simulink model "ModeInt"  (R2018b)
settings: Solver=FixedStepDiscrete  StartTime=0.0  StopTime=10.0  FixedStep=0.01  RelTol=1e-3
undefined symbols (not defined in the file or in its folder): c, CmprtMdHMIReqTp1, e, IfVeSMSeStNumConfig, MdReqTp1
(part 3 of 4)

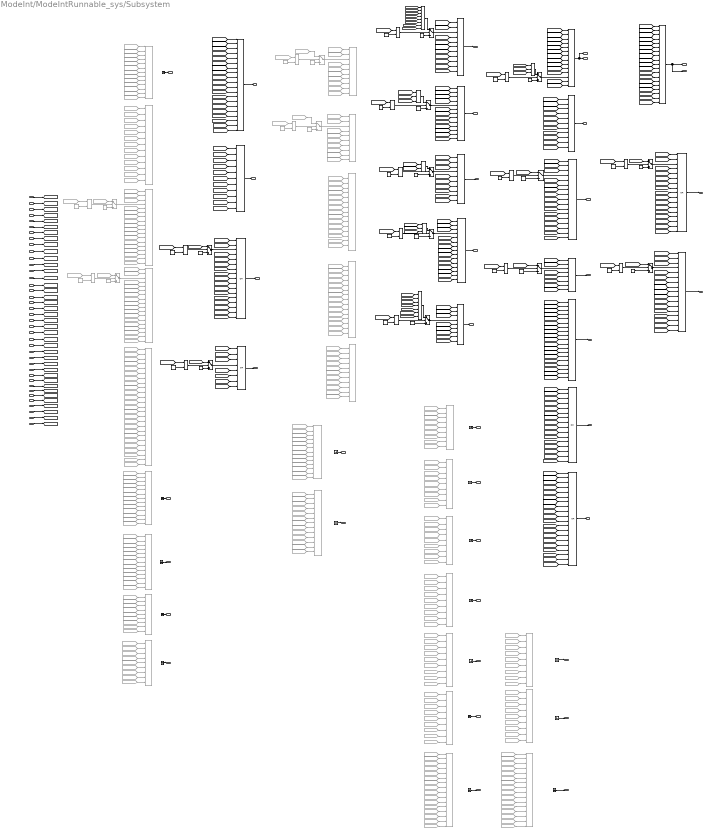
== system ModeInt/ModeIntRunnable_sys/Subsystem ==
  note: 2022-02-17:CR202175：修改需求506/548/551/552，新增需求712，完善座椅模式的打断策略。
  acsExtSoftInt : Inport
  acsEntySoftInt : Inport  Port=2
  LtVipSoftInt : Inport  Port=3
  RtVipSoftInt : Inport  Port=4
  LtLugSoftInt : Inport  Port=5
  RtLugSoftInt : Inport  Port=6
  AllLugSoftInt : Inport  Port=7
  LtRcvySoftInt : Inport  Port=8
  RtRcvySoftInt : Inport  Port=9
  SeStNumConfig : Inport  Port=10
  AllVipSoftInt : Inport  Port=11
  LtFamilySoftInt : Inport  Port=12
  RtFamilySoftInt : Inport  Port=13
  IntimacyLtSoftInt : Inport  Port=14
  IntimacyRtSoftInt : Inport  Port=15
  LtLyingSoftInt : Inport  Port=16
  RtLyingSoftInt : Inport  Port=17
  LgrstOpenLtSoftInt : Inport  Port=18
  LgrstCloseLtSoftInt : Inport  Port=19
  LgrstOpenRtSoftInt : Inport  Port=20
  LgrstCloseRtSoftInt : Inport  Port=21
  acsEntry4s2LSoftInt : Inport  Port=22
  " acsEntry4s2RSoftInt" : Inport  Port=23
  acsExit4s2LSoftInt : Inport  Port=24
  acsExit4s2RSoftInt : Inport  Port=25
  acsEntryAll4sBwdSoftInt : Inport  Port=26
  acsEntryAll4sFwdSoftInt : Inport  Port=27
  PasReclinerEntrySoftInt : Inport  Port=28
  PasReclinerExitSoftInt : Inport  Port=29
  VIPLtOutSoftInt : Inport  Port=30
  VIPRtOutSoftInt : Inport  Port=31
  VIPAllOutSoftInt : Inport  Port=32
  Big4SeatSoftInt : Inport  Port=33
  Unfold3LSoftInt : Inport  Port=34
  Unfold3RSoftInt : Inport  Port=35
  ExVIPRSoftInt : Inport  Port=36
  ExVIPROutSoftInt : Inport  Port=37
  WholeVehMem1SoftInt : Inport  Port=38
  WholeVehMem2SoftInt : Inport  Port=39
  Constant{1,3,5,7} (4 alike) : Constant  Commented=on  Value=IfVeSMSeStNumConfig.SeatNum7Config  OutDataTypeStr=Enum: IfVeSMSeStNumConfig
  Constant{10,12,14,16,18,20,22,24,26,28,30,32} (12 alike) : Constant  Value=0  OutDataTypeStr=uint8
  Constant{9,11,13,15,17,19,21,23,25,27,29,31} (12 alike) : Constant  Value=IfVeSMSeStNumConfig.SeatNum7Config  OutDataTypeStr=Enum: IfVeSMSeStNumConfig
  Constant{2,4,6,8} (4 alike) : Constant  Commented=on  Value=0  OutDataTypeStr=uint8
  Equal{1..4} (4 alike) : RelationalOperator  Commented=on  Operator===  OutDataTypeStr=boolean  RndMeth=Simplest
  Equal{5..16} (12 alike) : RelationalOperator  Operator===  OutDataTypeStr=boolean  RndMeth=Simplest
  From{,164,200,204,236,297,306,320,336} (9 alike) : From  Commented=on  GotoTag=LgrstOpenRtSoftInt
  From{1,6,16,22,27,31,34,37,87,99,119,131,170} (13 alike) : From  Commented=on  GotoTag=acsEntySoftInt
  From{10,17,23,43,138,155,181,185,194,197} (10 alike) : From  Commented=on  GotoTag=LtLugSoftInt
  From{2,8,28,32,38,88,97,100,109,120,122,146,206,228,275,284,311,327} (18 alike) : From  Commented=on  GotoTag=LtVipSoftInt
  From{3,9,29,35,39,42,101,110,136,147,171,180,216,240,293,302,313,328} (18 alike) : From  Commented=on  GotoTag=RtVipSoftInt
  From{4,13,20,91,102,111,123,150,172,177,235,277,286,314,330} (15 alike) : From  Commented=on  GotoTag=LtRcvySoftInt
  From{5,14,26,90,103,112,137,151,173,223,247,295,304,315,331} (15 alike) : From  Commented=on  GotoTag=RtRcvySoftInt
  From{47,53,67..70,73,76,81,93,104,113,174,205,207..208,210..212,276,285,294,303,312,329} (25 alike) : From  Commented=on  GotoTag=AllVipSoftInt
  From{55,75,79,84,105,114,145,148,154,156,158,162,188} (13 alike) : From  Commented=on  GotoTag=IntimacyLtSoftInt
  From{49,54,58,62,66,72,78,83,95,106,128,144,176} (13 alike) : From  Commented=on  GotoTag=RtFamilySoftInt
  From{50,59,96,107,125,149,157,159,163,167,179,184,189} (13 alike) : From  Commented=on  GotoTag=IntimacyRtSoftInt
  From{48,57,61,65,71,77,82,94,108,115,127,143,175} (13 alike) : From  Commented=on  GotoTag=LtFamilySoftInt
  From{11,18,24,45,139,153,182,186,195,198} (10 alike) : From  Commented=on  GotoTag=RtLugSoftInt
  From{36,40,44,117} (4 alike) : From  Commented=on  GotoTag=SeStNumConfig
  From{7,15,21,30,33,41,52,86,92,98,118,130,152} (13 alike) : From  Commented=on  GotoTag=acsExtSoftInt
  From{12,19,25,46,74,124,140,183,187,196,199} (11 alike) : From  Commented=on  GotoTag=AllLugSoftInt
  From{126,134,168,218,226,232,239,246,250,254,258,282,291,300,309,342} (16 alike) : From  Commented=on  GotoTag=acsEntryAll4sBwdSoftInt
  From{129,135,169,220,227,233,241,245,251,255,259,283,292,301,310,325} (16 alike) : From  Commented=on  GotoTag=acsEntryAll4sFwdSoftInt
  From{132,213,221,234,248,252,290,322,338} (9 alike) : From  Commented=on  GotoTag=acsEntry4s2LSoftInt
  From{133,214,222,238,249,253,281,324,340} (9 alike) : From  Commented=on  GotoTag=acsExit4s2LSoftInt
  From{141,215,229,242,256,260,308,323,339} (9 alike) : From  Commented=on  GotoTag=acsEntry4s2RSoftInt
  From{142,217,230,244,257,261,299,326,341} (9 alike) : From  Commented=on  GotoTag=acsExit4s2RSoftInt
  From{63,160,192,202,225,279,288,318,334} (9 alike) : From  Commented=on  GotoTag=LgrstOpenLtSoftInt
  From{161,166,193,203,224,280,289,319,335} (9 alike) : From  Commented=on  GotoTag=LgrstCloseLtSoftInt
  From{89,165,191,201,237,298,307,321,337} (9 alike) : From  Commented=on  GotoTag=LgrstCloseRtSoftInt
  From{60,80,178,209,231,278,287,316,332} (9 alike) : From  Commented=on  GotoTag=LtLyingSoftInt
  From{64,85,190,219,243,296,305,317,333} (9 alike) : From  Commented=on  GotoTag=RtLyingSoftInt
  Ground{,1..16} (17 alike) : Ground
  OR{,1,9..11,15} (6 alike) : Logic  Commented=on  Operator=OR  Inputs=13  AllPortsSameDT=off  OutDataTypeStr=boolean
  OR{12..13,16..23} (10 alike) : Logic  Commented=on  Operator=OR  Inputs=9  AllPortsSameDT=off  OutDataTypeStr=boolean
  OR14 : Logic  Commented=on  Operator=OR  Inputs=25  AllPortsSameDT=off  OutDataTypeStr=boolean
  OR2 : Logic  Commented=on  Operator=OR  Inputs=18  AllPortsSameDT=off  OutDataTypeStr=boolean
  OR24 : Logic  Commented=on  Operator=OR  Inputs=16  AllPortsSameDT=off  OutDataTypeStr=boolean
  OR25 : Logic  Commented=on  Operator=OR  Inputs=16  AllPortsSameDT=off  OutDataTypeStr=boolean
  OR26 : Logic  Operator=OR  Inputs=20  AllPortsSameDT=off  OutDataTypeStr=boolean
  OR27 : Logic  Operator=OR  Inputs=11  AllPortsSameDT=off  OutDataTypeStr=boolean
  OR28 : Logic  Operator=OR  Inputs=19  AllPortsSameDT=off  OutDataTypeStr=boolean
  OR{29,43,46..47} (4 alike) : Logic  Operator=OR  Inputs=17  AllPortsSameDT=off  OutDataTypeStr=boolean
  OR3 : Logic  Commented=on  Operator=OR  Inputs=18  AllPortsSameDT=off  OutDataTypeStr=boolean
  OR30 : Logic  Operator=OR  Inputs=8  AllPortsSameDT=off  OutDataTypeStr=boolean
  OR31 : Logic  Operator=OR  Inputs=8  AllPortsSameDT=off  OutDataTypeStr=boolean
  OR32 : Logic  Operator=OR  Inputs=11  AllPortsSameDT=off  OutDataTypeStr=boolean
  OR33 : Logic  Operator=OR  Inputs=13  AllPortsSameDT=off  OutDataTypeStr=boolean
  OR34 : Logic  Operator=OR  AllPortsSameDT=off  OutDataTypeStr=boolean
  OR35 : Logic  Operator=OR  Inputs=10  AllPortsSameDT=off  OutDataTypeStr=boolean
  OR36 : Logic  Operator=OR  Inputs=15  AllPortsSameDT=off  OutDataTypeStr=boolean
  OR37 : Logic  Operator=OR  Inputs=3  AllPortsSameDT=off  OutDataTypeStr=boolean
  OR38 : Logic  Operator=OR  Inputs=7  AllPortsSameDT=off  OutDataTypeStr=boolean
  OR39 : Logic  Operator=OR  Inputs=9  AllPortsSameDT=off  OutDataTypeStr=boolean
  OR4 : Logic  Commented=on  Operator=OR  Inputs=10  AllPortsSameDT=off  OutDataTypeStr=boolean
  OR40 : Logic  Operator=OR  Inputs=14  AllPortsSameDT=off  OutDataTypeStr=boolean
  OR41 : Logic  Operator=OR  Inputs=11  AllPortsSameDT=off  OutDataTypeStr=boolean
  OR42 : Logic  Operator=OR  Inputs=16  AllPortsSameDT=off  OutDataTypeStr=boolean
  OR44 : Logic  Operator=OR  Inputs=20  AllPortsSameDT=off  OutDataTypeStr=boolean
  OR45 : Logic  Operator=OR  Inputs=8  AllPortsSameDT=off  OutDataTypeStr=boolean
  OR48 : Logic  Operator=OR  Inputs=3  AllPortsSameDT=off  OutDataTypeStr=boolean
  OR49 : Logic  Operator=OR  Inputs=19  AllPortsSameDT=off  OutDataTypeStr=boolean
  OR5 : Logic  Commented=on  Operator=OR  Inputs=15  AllPortsSameDT=off  OutDataTypeStr=boolean
  OR50 : Logic  Operator=OR  Inputs=3  AllPortsSameDT=off  OutDataTypeStr=boolean
  OR6 : Logic  Commented=on  Operator=OR  Inputs=15  AllPortsSameDT=off  OutDataTypeStr=boolean
  OR7 : Logic  Commented=on  Operator=OR  Inputs=11  AllPortsSameDT=off  OutDataTypeStr=boolean
  OR8 : Logic  Commented=on  Operator=OR  Inputs=10  AllPortsSameDT=off  OutDataTypeStr=boolean
  Switch{1..4} (4 alike) : Switch  Commented=on  Criteria=u2 > Threshold
  Switch{5..16} (12 alike) : Switch  Criteria=u2 > Threshold
  SoftIntAcsExt : Outport
  SoftIntAcsEnty : Outport  Port=2
  SoftIntLfVip : Outport  Port=3
  SoftIntRtVip : Outport  Port=4
  SoftIntAllVip : Outport  Port=5
  SoftIntLfLug : Outport  Port=6
  SoftIntRtLug : Outport  Port=7
  SoftIntLfRcvy : Outport  Port=8
  SoftIntRtRcvy : Outport  Port=9
  SoftIntAllLug : Outport  Port=10
  SoftIntIntimacyLt : Outport  Port=11
  SoftIntIntimacyRt : Outport  Port=12
  SoftIntLtFamily : Outport  Port=13
  SoftIntLtLying : Outport  Port=14
  SoftIntRtFamily : Outport  Port=15
  SoftIntRtLying : Outport  Port=16
  SoftIntLgrstOpenLt : Outport  Port=17
  SoftIntLgrstCloseLt : Outport  Port=18
  SoftIntLgrstOpenRt : Outport  Port=19
  SoftIntLgrstCloseRt : Outport  Port=20
  SoftIntAcsEntry4s2L : Outport  Port=21
  SoftIntAcsExit4s2L : Outport  Port=22
  SoftIntAcsEntry4s2R : Outport  Port=23
  SoftIntAcsExit4s2R : Outport  Port=24
  SoftIntAcsEntryAll4sBwd : Outport  Port=25
  SoftIntAcsEntryAll4sFwd : Outport  Port=26
  SoftIntPasReclinerEntry : Outport  Port=27
  SoftIntPasReclinerExit : Outport  Port=28
  SoftIntVIPLtOut : Outport  Port=29
  SoftIntVIPRtOut : Outport  Port=30
  SoftIntVIPAllOut : Outport  Port=31
  SoftIntUnfold3L : Outport  Port=32
  SoftIntUnfold3R : Outport  Port=33
  SoftIntBig4Seat : Outport  Port=34
  SoftIntExVIPR : Outport  Port=35
  SoftIntExVIPROut : Outport  Port=36
  SoftIntWholeVehMem1 : Outport  Port=37
  SoftIntWholeVehMem2 : Outport  Port=38
  wires:
  acsExtSoftInt/1 -> [acsExtSoftInt]
  acsEntySoftInt/1 -> [acsEntySoftInt]
  LtVipSoftInt/1 -> [LtVipSoftInt]
  RtVipSoftInt/1 -> [RtVipSoftInt]
  LtLugSoftInt/1 -> [LtLugSoftInt]
  RtLugSoftInt/1 -> [RtLugSoftInt]
  AllLugSoftInt/1 -> [AllLugSoftInt]
  RtRcvySoftInt/1 -> [RtRcvySoftInt]
  LtRcvySoftInt/1 -> [LtRcvySoftInt]
  From15/1 -> OR2/1
  From16/1 -> OR2/2
  From17/1 -> OR2/3
  From19/1 -> OR2/5
  From20/1 -> OR2/6
  From21/1 -> OR3/1
  From22/1 -> OR3/2
  From24/1 -> OR3/4
  From25/1 -> OR3/5
  From26/1 -> OR3/6
  From27/1 -> OR4/1
  From31/1 -> OR5/2
  From30/1 -> OR5/1
  From1/1 -> OR/1
  From2/1 -> OR/2
  From3/1 -> OR/3
  From4/1 -> OR/4
  From5/1 -> OR/5
  From7/1 -> OR1/1
  From8/1 -> OR1/2
  From9/1 -> OR1/3
  From10/1 -> OR1/4
  From13/1 -> OR1/7
  From14/1 -> OR1/8
  From12/1 -> OR1/6
  From11/1 -> OR1/5
  SeStNumConfig/1 -> [SeStNumConfig]
  From23/1 -> Switch1/1
  Equal1/1 -> Switch1/2
  Constant2/1 -> Switch1/3
  From36/1 -> Equal1/1
  Constant1/1 -> Equal1/2
  Switch1/1 -> OR3/3
  Equal2/1 -> Switch2/2
  Constant4/1 -> Switch2/3
  From40/1 -> Equal2/1
  Constant3/1 -> Equal2/2
  Switch2/1 -> OR4/3
  From6/1 -> OR8/1
  Constant5/1 -> Equal3/2
  From44/1 -> Equal3/1
  Constant6/1 -> Switch3/3
  Equal3/1 -> Switch3/2
  From46/1 -> OR/8
  From45/1 -> OR/7
  From43/1 -> OR/6
  AllVipSoftInt/1 -> [AllVipSoftInt]
  LtFamilySoftInt/1 -> [LtFamilySoftInt]
  RtFamilySoftInt/1 -> [RtFamilySoftInt]
  IntimacyLtSoftInt/1 -> [IntimacyLtSoftInt]
  LtLyingSoftInt/1 -> [LtLyingSoftInt]
  RtLyingSoftInt/1 -> [RtLyingSoftInt]
  From47/1 -> OR/9
  From48/1 -> OR/10
  From49/1 -> OR/11
  From70/1 -> OR1/9
  From71/1 -> OR1/10
  From72/1 -> OR1/11
  From98/1 -> OR10/1
  From99/1 -> OR10/2
  From100/1 -> OR10/3
  From101/1 -> OR10/4
  From102/1 -> OR10/5
  From103/1 -> OR10/6
  From104/1 -> OR10/7
  IntimacyRtSoftInt/1 -> [IntimacyRtSoftInt]
  LgrstCloseLtSoftInt/1 -> [LgrstCloseLtSoftInt]
  LgrstOpenLtSoftInt/1 -> [LgrstOpenLtSoftInt]
  LgrstOpenRtSoftInt/1 -> [LgrstOpenRtSoftInt]
  LgrstCloseRtSoftInt/1 -> [LgrstCloseRtSoftInt]
  From106/1 -> OR10/8
  From77/1 -> OR2/7
  From78/1 -> OR2/8
  From80/1 -> OR2/9
  From82/1 -> OR3/7
  From83/1 -> OR3/8
  From167/1 -> OR3/10
  From84/1 -> OR3/9
  From85/1 -> OR3/12
  From/1 -> OR3/13
  From89/1 -> OR3/14
  From145/1 -> OR14/8
  From179/1 -> OR14/9
  From144/1 -> OR14/7
  From143/1 -> OR14/6
  From140/1 -> OR14/5
  From130/1 -> OR14/1
  From131/1 -> OR14/2
  From138/1 -> OR14/3
  From139/1 -> OR14/4
  From148/1 -> OR/12
  From149/1 -> OR/13
  From154/1 -> OR1/12
  From50/1 -> OR1/13
  From105/1 -> OR10/9
  From189/1 -> OR10/10
  From197/1 -> OR10/11
  From198/1 -> OR10/12
  From199/1 -> OR10/13
  From118/1 -> OR11/1
  From119/1 -> OR11/2
  From109/1 -> OR11/3
  From110/1 -> OR11/4
  From113/1 -> OR11/5
  From111/1 -> OR11/6
  From112/1 -> OR11/7
  From115/1 -> OR11/8
  From114/1 -> OR11/9
  From184/1 -> OR11/10
  From194/1 -> OR11/11
  From195/1 -> OR11/12
  From196/1 -> OR11/13
  From122/1 -> OR12/1
  From136/1 -> OR13/1
  From29/1 -> Switch2/1
  From52/1 -> OR4/2
  From28/1 -> OR4/4
  From53/1 -> OR4/5
  Constant7/1 -> Equal4/2
  From117/1 -> Equal4/1
  Constant8/1 -> Switch4/3
  Equal4/1 -> Switch4/2
  From18/1 -> Switch4/1
  Switch4/1 -> OR2/4
  From120/1 -> Switch3/1
  From74/1 -> OR4/6
  From75/1 -> OR4/7
  From107/1 -> OR4/8
  From108/1 -> OR4/9
  From54/1 -> OR4/10
  From41/1 -> OR8/2
  Switch3/1 -> OR8/3
  From42/1 -> OR8/4
  From73/1 -> OR8/5
  From124/1 -> OR8/6
  From125/1 -> OR8/8
  From55/1 -> OR8/7
  From60/1 -> OR5/9
  From161/1 -> OR5/11
  From160/1 -> OR5/10
  From34/1 -> OR6/1
  From33/1 -> OR6/2
  From146/1 -> OR14/10
  From147/1 -> OR14/11
  From150/1 -> OR14/12
  From151/1 -> OR14/13
  From37/1 -> OR7/1
  From152/1 -> OR7/2
  From38/1 -> OR7/3
  From39/1 -> OR7/4
  From69/1 -> OR7/5
  From155/1 -> OR7/6
  From153/1 -> OR7/7
  From65/1 -> OR7/8
  From66/1 -> OR7/9
  From156/1 -> OR7/10
  From157/1 -> OR7/11
  From87/1 -> OR9/1
  From86/1 -> OR9/2
  From88/1 -> OR9/3
  From180/1 -> OR9/4
  From93/1 -> OR9/5
  From182/1 -> OR9/7
  From181/1 -> OR9/6
  From183/1 -> OR9/8
  From94/1 -> OR9/9
  From95/1 -> OR9/10
  From91/1 -> OR9/11
  From90/1 -> OR9/12
  From96/1 -> OR9/13
  From170/1 -> OR15/1
  From92/1 -> OR15/2
  From97/1 -> OR15/3
  From171/1 -> OR15/4
  From174/1 -> OR15/5
  From185/1 -> OR15/6
  From186/1 -> OR15/7
  From187/1 -> OR15/8
  From175/1 -> OR15/9
  From176/1 -> OR15/10
  From188/1 -> OR15/11
  From173/1 -> OR15/13
  From177/1 -> OR15/12
  From206/1 -> OR16/1
  From228/1 -> OR18/1
  From216/1 -> OR17/1
  From240/1 -> OR19/1
  From79/1 -> OR2/10
  From59/1 -> OR2/11
  From63/1 -> OR2/12
  From166/1 -> OR2/13
  From76/1 -> OR2/14
  From81/1 -> OR3/11
  From178/1 -> OR14/14
  From190/1 -> OR14/15
  From192/1 -> OR14/16
  From193/1 -> OR14/17
  From204/1 -> OR14/18
  From191/1 -> OR14/19
  From203/1 -> OR12/5
  From202/1 -> OR12/4
  From123/1 -> OR12/3
  From205/1 -> OR12/2
  From201/1 -> OR13/5
  From200/1 -> OR13/4
  From137/1 -> OR13/3
  From207/1 -> OR13/2
  From208/1 -> OR16/2
  From209/1 -> OR16/3
  From172/1 -> OR16/4
  From224/1 -> OR16/5
  From210/1 -> OR18/2
  From231/1 -> OR18/3
  From235/1 -> OR18/4
  From225/1 -> OR18/5
  From237/1 -> OR17/5
  From223/1 -> OR17/4
  From219/1 -> OR17/3
  From211/1 -> OR17/2
  From236/1 -> OR19/5
  From247/1 -> OR19/4
  From243/1 -> OR19/3
  From212/1 -> OR19/2
  From127/1 -> OR8/9
  From128/1 -> OR8/10
  From32/1 -> OR5/3
  From67/1 -> OR5/4
  From57/1 -> OR5/5
  From58/1 -> OR5/6
  From158/1 -> OR5/7
  From159/1 -> OR5/8
  From35/1 -> OR6/3
  From68/1 -> OR6/4
  From61/1 -> OR6/5
  From62/1 -> OR6/6
  From162/1 -> OR6/7
  From163/1 -> OR6/8
  From64/1 -> OR6/9
  From164/1 -> OR6/10
  From165/1 -> OR6/11
  acsEntry4s2LSoftInt/1 -> [acsEntry4s2LSoftInt]
  " acsEntry4s2RSoftInt"/1 -> [acsEntry4s2RSoftInt]
  acsExit4s2LSoftInt/1 -> [acsExit4s2LSoftInt]
  acsExit4s2RSoftInt/1 -> [acsExit4s2RSoftInt]
  acsEntryAll4sBwdSoftInt/1 -> [acsEntryAll4sBwdSoftInt]
  acsEntryAll4sFwdSoftInt/1 -> [acsEntryAll4sFwdSoftInt]
  From132/1 -> OR2/15
  From133/1 -> OR2/16
  From134/1 -> OR2/17
  From135/1 -> OR2/18
  From141/1 -> OR3/15
  From142/1 -> OR3/16
  From168/1 -> OR3/17
  From169/1 -> OR3/18
  From213/1 -> OR14/20
  From214/1 -> OR14/21
  From215/1 -> OR14/22
  From217/1 -> OR14/23
  From218/1 -> OR14/24
  From220/1 -> OR14/25
  From221/1 -> OR12/6
  From222/1 -> OR12/7
  From226/1 -> OR12/8
  From227/1 -> OR12/9
  From229/1 -> OR13/6
  From230/1 -> OR13/7
  From232/1 -> OR13/8
  From233/1 -> OR13/9
  From234/1 -> OR5/12
  From238/1 -> OR5/13
  From239/1 -> OR5/14
  From241/1 -> OR5/15
  From242/1 -> OR6/12
  From244/1 -> OR6/13
  From246/1 -> OR6/14
  From245/1 -> OR6/15
  From248/1 -> OR16/6
  From249/1 -> OR16/7
  From250/1 -> OR16/8
  From251/1 -> OR16/9
  From252/1 -> OR18/6
  From253/1 -> OR18/7
  From254/1 -> OR18/8
  From255/1 -> OR18/9
  From256/1 -> OR17/6
  From257/1 -> OR17/7
  From258/1 -> OR17/8
  From259/1 -> OR17/9
  From260/1 -> OR19/6
  From261/1 -> OR19/7
  From126/1 -> OR19/8
  From129/1 -> OR19/9
  From275/1 -> OR20/1
  From276/1 -> OR20/2
  From277/1 -> OR20/3
  From278/1 -> OR20/4
  From279/1 -> OR20/5
  From280/1 -> OR20/6
  From281/1 -> OR20/7
  From282/1 -> OR20/8
  From283/1 -> OR20/9
  From287/1 -> OR21/4
  From286/1 -> OR21/3
  From285/1 -> OR21/2
  From284/1 -> OR21/1
  From289/1 -> OR21/6
  From288/1 -> OR21/5
  From290/1 -> OR21/7
  From291/1 -> OR21/8
  From292/1 -> OR21/9
  From293/1 -> OR22/1
  From294/1 -> OR22/2
  From295/1 -> OR22/3
  From296/1 -> OR22/4
  From298/1 -> OR22/6
  From297/1 -> OR22/5
  From299/1 -> OR22/7
  From300/1 -> OR22/8
  From301/1 -> OR22/9
  From302/1 -> OR23/1
  From303/1 -> OR23/2
  From304/1 -> OR23/3
  From305/1 -> OR23/4
  From306/1 -> OR23/5
  From307/1 -> OR23/6
  From308/1 -> OR23/7
  From310/1 -> OR23/9
  From309/1 -> OR23/8
  From311/1 -> OR24/1
  From313/1 -> OR24/2
  From312/1 -> OR24/3
  From314/1 -> OR24/4
  From315/1 -> OR24/5
  From316/1 -> OR24/6
  From317/1 -> OR24/7
  From318/1 -> OR24/8
  From319/1 -> OR24/9
  From320/1 -> OR24/10
  From321/1 -> OR24/11
  From323/1 -> OR24/14
  From324/1 -> OR24/13
  From326/1 -> OR24/15
  From322/1 -> OR24/12
  From325/1 -> OR24/16
  From327/1 -> OR25/1
  From328/1 -> OR25/2
  From329/1 -> OR25/3
  From330/1 -> OR25/4
  From331/1 -> OR25/5
  From332/1 -> OR25/6
  From333/1 -> OR25/7
  From334/1 -> OR25/8
  From335/1 -> OR25/9
  From336/1 -> OR25/10
  From337/1 -> OR25/11
  From338/1 -> OR25/12
  From339/1 -> OR25/14
  From340/1 -> OR25/13
  From341/1 -> OR25/15
  From342/1 -> OR25/16
  PasReclinerEntrySoftInt/1 -> [PasReclinerEntrySoftInt]
  PasReclinerExitSoftInt/1 -> [PasReclinerExitSoftInt]
  VIPLtOutSoftInt/1 -> [VIPLtOutSoftInt]
  VIPRtOutSoftInt/1 -> [VIPRtOutSoftInt]
  VIPAllOutSoftInt/1 -> [VIPAllOutSoftInt]
  Ground/1 -> SoftIntAcsExt/1
  Ground1/1 -> SoftIntLtFamily/1
  Ground2/1 -> SoftIntRtFamily/1
  Ground3/1 -> SoftIntLtLying/1
  Ground4/1 -> SoftIntRtLying/1
  Ground5/1 -> SoftIntIntimacyLt/1
  Ground6/1 -> SoftIntIntimacyRt/1
  Ground7/1 -> SoftIntLgrstOpenLt/1
  Ground8/1 -> SoftIntLgrstCloseLt/1
  Ground9/1 -> SoftIntLgrstOpenRt/1
  Ground10/1 -> SoftIntLgrstCloseRt/1
  Ground11/1 -> SoftIntAcsEntry4s2L/1
  Ground12/1 -> SoftIntAcsExit4s2L/1
  Ground13/1 -> SoftIntAcsEntryAll4sBwd/1
  Ground14/1 -> SoftIntAcsEntry4s2R/1
  Ground15/1 -> SoftIntAcsExit4s2R/1
  Ground16/1 -> SoftIntAcsEntryAll4sFwd/1
  [LtVipSoftInt] -> OR26/1
  [RtVipSoftInt] -> OR26/2
  [LtLugSoftInt] -> OR26/3
  [RtLugSoftInt] -> OR26/4
  [AllLugSoftInt] -> OR26/5
  [LtRcvySoftInt] -> OR26/6
  [RtRcvySoftInt] -> OR26/7
  [VIPAllOutSoftInt] -> OR26/11
  [VIPRtOutSoftInt] -> OR26/10
  [VIPLtOutSoftInt] -> OR26/9
  [AllVipSoftInt] -> OR26/8
  OR26/1 -> SoftIntAcsEnty/1
  [acsEntySoftInt] -> OR27/1
  OR27/1 -> SoftIntLfVip/1
  Constant11/1 -> Equal6/2
  [SeStNumConfig] -> Equal6/1
  Constant12/1 -> Switch6/3
  Equal6/1 -> Switch6/2
  [acsEntySoftInt] -> OR29/1
  [AllVipSoftInt] -> OR29/2
  Switch6/1 -> OR29/3
  [RtLugSoftInt] -> OR29/4
  [AllLugSoftInt] -> OR29/5
  [RtRcvySoftInt] -> OR29/6
  [PasReclinerEntrySoftInt] -> OR29/7
  [PasReclinerExitSoftInt] -> OR29/8
  [VIPRtOutSoftInt] -> OR29/9
  [VIPAllOutSoftInt] -> OR29/10
  OR29/1 -> SoftIntRtVip/1
  [acsEntySoftInt] -> OR30/1
  OR30/1 -> SoftIntAllVip/1
  Constant13/1 -> Equal7/2
  [SeStNumConfig] -> Equal7/1
  Constant14/1 -> Switch7/3
  Equal7/1 -> Switch7/2
  [RtVipSoftInt] -> OR31/1
  [VIPRtOutSoftInt] -> OR31/2
  OR31/1 -> Switch7/1
  [acsEntySoftInt] -> OR32/1
  [LtVipSoftInt] -> OR32/2
  Switch7/1 -> OR32/3
  [AllVipSoftInt] -> OR32/4
  [AllLugSoftInt] -> OR32/5
  [VIPLtOutSoftInt] -> OR32/6
  [VIPAllOutSoftInt] -> OR32/7
  OR32/1 -> SoftIntLfLug/1
  Equal8/1 -> Switch8/2
  Constant16/1 -> Switch8/3
  [SeStNumConfig] -> Equal8/1
  Constant15/1 -> Equal8/2
  [acsEntySoftInt] -> OR33/1
  [RtVipSoftInt] -> OR33/2
  [AllVipSoftInt] -> OR33/3
  [AllLugSoftInt] -> OR33/4
  Switch8/1 -> OR33/5
  [VIPRtOutSoftInt] -> OR33/6
  [VIPAllOutSoftInt] -> OR33/7
  OR33/1 -> SoftIntRtLug/1
  Constant17/1 -> Equal9/2
  [SeStNumConfig] -> Equal9/1
  Constant18/1 -> Switch9/3
  Equal9/1 -> Switch9/2
  [AllLugSoftInt] -> OR34/2
  [LtLugSoftInt] -> OR34/1
  OR34/1 -> Switch9/1
  [VIPAllOutSoftInt] -> OR35/6
  [VIPLtOutSoftInt] -> OR35/5
  Switch9/1 -> OR35/4
  [AllVipSoftInt] -> OR35/3
  [LtVipSoftInt] -> OR35/2
  [acsEntySoftInt] -> OR35/1
  OR35/1 -> SoftIntLfRcvy/1
  Constant21/1 -> Equal11/2
  [SeStNumConfig] -> Equal11/1
  Constant22/1 -> Switch11/3
  Equal11/1 -> Switch11/2
  [LtLugSoftInt] -> OR37/1
  OR37/1 -> Switch11/1
  [AllLugSoftInt] -> OR37/3
  [RtLugSoftInt] -> OR37/2
  [VIPAllOutSoftInt] -> OR36/6
  [VIPRtOutSoftInt] -> OR36/5
  Switch11/1 -> OR36/4
  [AllVipSoftInt] -> OR36/3
  [RtVipSoftInt] -> OR36/2
  [acsEntySoftInt] -> OR36/1
  OR36/1 -> SoftIntRtRcvy/1
  OR38/1 -> Switch10/1
  Equal10/1 -> Switch10/2
  Constant20/1 -> Switch10/3
  [SeStNumConfig] -> Equal10/1
  Constant19/1 -> Equal10/2
  [LtRcvySoftInt] -> OR31/3
  [RtRcvySoftInt] -> OR31/4
  [acsEntySoftInt] -> OR39/1
  OR39/1 -> SoftIntAllLug/1
  OR40/1 -> SoftIntPasReclinerExit/1, SoftIntPasReclinerEntry/1
  [acsEntySoftInt] -> OR41/1
  [AllVipSoftInt] -> OR41/3
  [LtVipSoftInt] -> OR41/2
  OR41/1 -> SoftIntVIPLtOut/1
  Equal13/1 -> Switch13/2
  Constant26/1 -> Switch13/3
  [SeStNumConfig] -> Equal13/1
  Constant25/1 -> Equal13/2
  [LtLugSoftInt] -> Switch13/1
  [acsEntySoftInt] -> OR43/1
  [RtVipSoftInt] -> OR43/2
  [AllVipSoftInt] -> OR43/3
  [RtRcvySoftInt] -> OR43/5
  Switch13/1 -> OR43/4
  [RtLugSoftInt] -> OR43/6
  [AllLugSoftInt] -> OR43/7
  [VIPAllOutSoftInt] -> OR43/8
  [PasReclinerEntrySoftInt] -> OR43/9
  [PasReclinerExitSoftInt] -> OR43/10
  OR43/1 -> SoftIntVIPRtOut/1
  Constant27/1 -> Equal14/2
  [SeStNumConfig] -> Equal14/1
  Constant28/1 -> Switch14/3
  Equal14/1 -> Switch14/2
  [acsEntySoftInt] -> OR45/1
  [AllVipSoftInt] -> OR45/2
  Switch14/1 -> OR45/3
  [AllLugSoftInt] -> OR45/4
  OR45/1 -> SoftIntVIPAllOut/1
  [RtVipSoftInt] -> OR38/1
  [RtRcvySoftInt] -> OR38/2
  Switch10/1 -> OR39/4
  [AllVipSoftInt] -> OR39/3
  [VIPAllOutSoftInt] -> OR39/2
  [AllLugSoftInt] -> OR30/2
  [VIPAllOutSoftInt] -> OR30/3
  [LtLugSoftInt] -> OR27/2
  [AllLugSoftInt] -> OR27/3
  [LtRcvySoftInt] -> OR27/4
  [AllVipSoftInt] -> OR27/5
  [VIPLtOutSoftInt] -> OR27/6
  [VIPAllOutSoftInt] -> OR27/7
  [LtLugSoftInt] -> Switch6/1
  [VIPAllOutSoftInt] -> OR41/7
  [AllLugSoftInt] -> OR41/6
  [LtLugSoftInt] -> OR41/5
  [LtRcvySoftInt] -> OR41/4
  [LtLugSoftInt] -> Switch14/1
  Big4SeatSoftInt/1 -> [Big4SeatSoftInt]
  Unfold3LSoftInt/1 -> [Unfold3LSoftInt]
  Unfold3RSoftInt/1 -> [Unfold3RSoftInt]
  [Unfold3LSoftInt] -> OR26/12
  [Big4SeatSoftInt] -> OR26/14
  [Unfold3RSoftInt] -> OR26/13
  [Unfold3LSoftInt] -> OR27/8
  [Big4SeatSoftInt] -> OR27/9
  [Unfold3LSoftInt] -> OR29/11
  [Unfold3RSoftInt] -> OR29/12
  [Big4SeatSoftInt] -> OR29/13
  Constant9/1 -> Equal5/2
  Constant10/1 -> Switch5/3
  [SeStNumConfig] -> Equal5/1
  Equal5/1 -> Switch5/2
  [LtLugSoftInt] -> Switch5/1
  Switch5/1 -> OR30/4
  [Unfold3LSoftInt] -> OR30/5
  [Big4SeatSoftInt] -> OR30/6
  [Unfold3LSoftInt] -> OR35/7
  [Big4SeatSoftInt] -> OR35/8
  [Unfold3LSoftInt] -> OR36/7
  [Unfold3RSoftInt] -> OR36/8
  [Big4SeatSoftInt] -> OR36/9
  [Unfold3LSoftInt] -> OR39/5
  [Unfold3RSoftInt] -> OR39/6
  [Big4SeatSoftInt] -> OR39/7
  [Unfold3LSoftInt] -> OR41/8
  [Big4SeatSoftInt] -> OR41/9
  [Unfold3LSoftInt] -> OR43/11
  [Unfold3RSoftInt] -> OR43/12
  [Big4SeatSoftInt] -> OR43/13
  [Unfold3LSoftInt] -> OR45/5
  [Big4SeatSoftInt] -> OR45/6
  [acsEntySoftInt] -> OR28/1
  [LtVipSoftInt] -> OR28/2
  [RtVipSoftInt] -> OR28/3
  [AllVipSoftInt] -> OR28/4
  [RtRcvySoftInt] -> OR28/6
  [LtLugSoftInt] -> OR28/7
  [RtLugSoftInt] -> OR28/8
  [AllLugSoftInt] -> OR28/9
  [VIPLtOutSoftInt] -> OR28/10
  [VIPRtOutSoftInt] -> OR28/11
  [VIPAllOutSoftInt] -> OR28/12
  [Big4SeatSoftInt] -> OR28/13
  OR28/1 -> SoftIntUnfold3L/1
  [LtRcvySoftInt] -> OR28/5
  [RtVipSoftInt] -> OR42/2
  [acsEntySoftInt] -> OR42/1
  [AllVipSoftInt] -> OR42/3
  [RtRcvySoftInt] -> OR42/4
  [LtLugSoftInt] -> OR42/5
  [RtLugSoftInt] -> OR42/6
  [AllLugSoftInt] -> OR42/7
  [VIPRtOutSoftInt] -> OR42/8
  [VIPAllOutSoftInt] -> OR42/9
  [Big4SeatSoftInt] -> OR42/10
  OR42/1 -> SoftIntUnfold3R/1
  [acsEntySoftInt] -> OR44/1
  [LtVipSoftInt] -> OR44/2
  [RtVipSoftInt] -> OR44/3
  [AllVipSoftInt] -> OR44/4
  [LtRcvySoftInt] -> OR44/5
  [RtRcvySoftInt] -> OR44/6
  [LtLugSoftInt] -> OR44/7
  [RtLugSoftInt] -> OR44/8
  [AllLugSoftInt] -> OR44/9
  [Unfold3LSoftInt] -> OR44/10
  [Unfold3RSoftInt] -> OR44/11
  [VIPLtOutSoftInt] -> OR44/12
  [VIPRtOutSoftInt] -> OR44/13
  [VIPAllOutSoftInt] -> OR44/14
  OR44/1 -> SoftIntBig4Seat/1
  ExVIPRSoftInt/1 -> [ExVIPRSoftInt]
  ExVIPROutSoftInt/1 -> [ExVIPROutSoftInt]
  [ExVIPRSoftInt] -> OR26/15
  [ExVIPROutSoftInt] -> OR26/16
  [ExVIPRSoftInt] -> OR29/14
  [ExVIPROutSoftInt] -> OR29/15
  [ExVIPRSoftInt] -> OR31/5
  [ExVIPROutSoftInt] -> OR31/6
  [ExVIPRSoftInt] -> OR36/10
  [ExVIPROutSoftInt] -> OR36/11
  [ExVIPRSoftInt] -> OR38/3
  [ExVIPROutSoftInt] -> OR38/5
  [VIPRtOutSoftInt] -> OR38/4
  [ExVIPROutSoftInt] -> OR43/15
  [ExVIPRSoftInt] -> OR43/14
  [ExVIPRSoftInt] -> OR28/14
  [ExVIPROutSoftInt] -> OR28/15
  [ExVIPRSoftInt] -> OR42/11
  [ExVIPROutSoftInt] -> OR42/12
  [ExVIPRSoftInt] -> OR44/15
  [ExVIPROutSoftInt] -> OR44/16
  [AllLugSoftInt] -> OR46/5
  [RtVipSoftInt] -> OR46/14
  Constant23/1 -> Equal12/2
  [LtLugSoftInt] -> Switch12/1
  [ExVIPROutSoftInt] -> OR46/15
  [Big4SeatSoftInt] -> OR46/13
  [SeStNumConfig] -> Equal12/1
  [PasReclinerEntrySoftInt] -> OR46/7
  Equal12/1 -> Switch12/2
  [acsEntySoftInt] -> OR46/1
  [Unfold3LSoftInt] -> OR46/11
  [Unfold3RSoftInt] -> OR46/12
  [VIPAllOutSoftInt] -> OR46/10
  [AllVipSoftInt] -> OR46/2
  Switch12/1 -> OR46/3
  [VIPRtOutSoftInt] -> OR46/9
  [RtLugSoftInt] -> OR46/4
  [RtRcvySoftInt] -> OR46/6
  [PasReclinerExitSoftInt] -> OR46/8
  Constant24/1 -> Switch12/3
  OR46/1 -> SoftIntExVIPR/1
  [AllVipSoftInt] -> OR47/3
  [Unfold3LSoftInt] -> OR47/11
  [SeStNumConfig] -> Equal15/1
  [Unfold3RSoftInt] -> OR47/12
  [Big4SeatSoftInt] -> OR47/13
  [RtVipSoftInt] -> OR47/2
  [AllLugSoftInt] -> OR47/7
  [PasReclinerEntrySoftInt] -> OR47/9
  [VIPAllOutSoftInt] -> OR47/8
  Constant29/1 -> Equal15/2
  Switch15/1 -> OR47/4
  [RtRcvySoftInt] -> OR47/5
  Equal15/1 -> Switch15/2
  Constant30/1 -> Switch15/3
  [RtLugSoftInt] -> OR47/6
  [acsEntySoftInt] -> OR47/1
  [PasReclinerExitSoftInt] -> OR47/10
  [VIPRtOutSoftInt] -> OR47/15
  [ExVIPRSoftInt] -> OR47/14
  [LtLugSoftInt] -> Switch15/1
  OR47/1 -> SoftIntExVIPROut/1
  [Unfold3RSoftInt] -> OR33/8
  [Big4SeatSoftInt] -> OR33/9
  [ExVIPRSoftInt] -> OR33/10
  [ExVIPROutSoftInt] -> OR33/11
  [Unfold3LSoftInt] -> OR32/8
  [Big4SeatSoftInt] -> OR32/9
  Constant31/1 -> Equal16/2
  Constant32/1 -> Switch16/3
  Equal16/1 -> Switch16/2
  [LtLugSoftInt] -> OR48/1
  [RtLugSoftInt] -> OR48/2
  [AllLugSoftInt] -> OR48/3
  OR48/1 -> Switch16/1
  [SeStNumConfig] -> Equal16/1
  [RtVipSoftInt] -> OR40/1
  [AllVipSoftInt] -> OR40/2
  [VIPRtOutSoftInt] -> OR40/3
  [VIPAllOutSoftInt] -> OR40/4
  [ExVIPRSoftInt] -> OR40/5
  [ExVIPROutSoftInt] -> OR40/6
  [acsEntySoftInt] -> OR40/7
  [Unfold3LSoftInt] -> OR40/8
  [Unfold3RSoftInt] -> OR40/9
  [RtRcvySoftInt] -> OR40/10
  [Big4SeatSoftInt] -> OR40/11
  Switch16/1 -> OR40/12
  WholeVehMem1SoftInt/1 -> [WholeVehMem1SoftInt]
  WholeVehMem2SoftInt/1 -> [WholeVehMem2SoftInt]
  [WholeVehMem1SoftInt] -> OR26/17
  [WholeVehMem2SoftInt] -> OR26/18
  [WholeVehMem1SoftInt] -> OR27/10
  [WholeVehMem2SoftInt] -> OR27/11
  [WholeVehMem1SoftInt] -> OR29/16
  [WholeVehMem2SoftInt] -> OR29/17
  [WholeVehMem1SoftInt] -> OR30/7
  [WholeVehMem2SoftInt] -> OR30/8
  [WholeVehMem1SoftInt] -> OR32/10
  [WholeVehMem2SoftInt] -> OR32/11
  [WholeVehMem1SoftInt] -> OR33/12
  [WholeVehMem2SoftInt] -> OR33/13
  [WholeVehMem1SoftInt] -> OR35/9
  [WholeVehMem2SoftInt] -> OR35/10
  [WholeVehMem1SoftInt] -> OR36/12
  [WholeVehMem2SoftInt] -> OR36/13
  [WholeVehMem1SoftInt] -> OR39/8
  [WholeVehMem2SoftInt] -> OR39/9
  [WholeVehMem1SoftInt] -> OR40/13
  [WholeVehMem2SoftInt] -> OR40/14
  [WholeVehMem1SoftInt] -> OR41/10
  [WholeVehMem2SoftInt] -> OR41/11
  [WholeVehMem1SoftInt] -> OR43/16
  [WholeVehMem2SoftInt] -> OR43/17
  [WholeVehMem1SoftInt] -> OR45/7
  [WholeVehMem2SoftInt] -> OR45/8
  [WholeVehMem1SoftInt] -> OR28/16
  [WholeVehMem2SoftInt] -> OR28/17
  [WholeVehMem1SoftInt] -> OR42/13
  [WholeVehMem2SoftInt] -> OR42/14
  [WholeVehMem1SoftInt] -> OR44/17
  [WholeVehMem2SoftInt] -> OR44/18
  [WholeVehMem1SoftInt] -> OR46/16
  [WholeVehMem2SoftInt] -> OR46/17
  [WholeVehMem1SoftInt] -> OR47/16
  [WholeVehMem2SoftInt] -> OR47/17
  [acsEntySoftInt] -> OR49/1
  [LtVipSoftInt] -> OR49/2
  [RtVipSoftInt] -> OR49/3
  [AllVipSoftInt] -> OR49/4
  [LtLugSoftInt] -> OR49/5
  [RtLugSoftInt] -> OR49/6
  [AllLugSoftInt] -> OR49/7
  [LtRcvySoftInt] -> OR49/8
  [RtRcvySoftInt] -> OR49/9
  [VIPLtOutSoftInt] -> OR49/10
  [VIPRtOutSoftInt] -> OR49/11
  [VIPAllOutSoftInt] -> OR49/12
  [Unfold3LSoftInt] -> OR49/13
  [Unfold3RSoftInt] -> OR49/14
  [Big4SeatSoftInt] -> OR49/15
  [PasReclinerExitSoftInt] -> OR49/18
  [PasReclinerEntrySoftInt] -> OR49/19
  [ExVIPRSoftInt] -> OR49/16
  [ExVIPROutSoftInt] -> OR49/17
  OR49/1 -> SoftIntWholeVehMem2/1, SoftIntWholeVehMem1/1
  [PasReclinerEntrySoftInt] -> OR26/19
  [PasReclinerExitSoftInt] -> OR26/20
  [PasReclinerEntrySoftInt] -> OR31/7
  [PasReclinerExitSoftInt] -> OR31/8
  [RtRcvySoftInt] -> OR50/1
  [PasReclinerEntrySoftInt] -> OR50/2
  OR50/1 -> Switch8/1
  [PasReclinerExitSoftInt] -> OR50/3
  [PasReclinerEntrySoftInt] -> OR36/14
  [PasReclinerExitSoftInt] -> OR36/15
  [PasReclinerEntrySoftInt] -> OR28/18
  [PasReclinerExitSoftInt] -> OR28/19
  [PasReclinerEntrySoftInt] -> OR42/15
  [PasReclinerExitSoftInt] -> OR42/16
  [PasReclinerEntrySoftInt] -> OR44/19
  [PasReclinerExitSoftInt] -> OR44/20
  [PasReclinerEntrySoftInt] -> OR38/6
  [PasReclinerExitSoftInt] -> OR38/7
